simulink model "test_lineestimator_simulink"  (R2015a)
settings: Solver=ode45  StartTime=0.0  StopTime=10.0  RelTol=1e-3
undefined symbols (not defined in the file): field_x, field_y
settings Model: Creator=tzwijger  LastModifiedBy=tzwijger

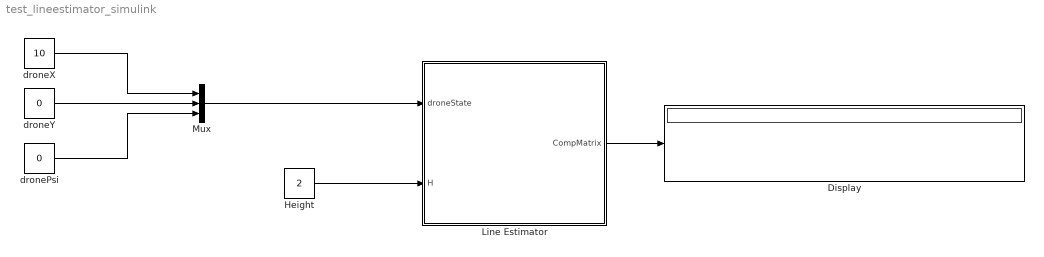
== system test_lineestimator_simulink ==
  Display : Display
  Height : Constant  Value=2
  Line Estimator : Subsystem
  Mux : Mux  Inputs=3
  dronePsi : Constant  Value=0
  droneX : Constant  Value=10
  droneY : Constant  Value=0
  wires:
  Mux/1 -> Line Estimator/1(droneState)
  droneX/1 -> Mux/1
  droneY/1 -> Mux/2
  dronePsi/1 -> Mux/3
  Height/1 -> Line Estimator/2(H)
  Line Estimator/1(CompMatrix) -> Display/1

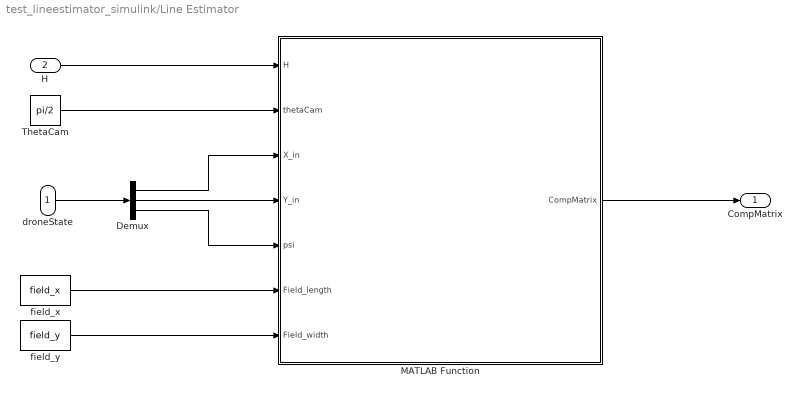
== system test_lineestimator_simulink/Line Estimator ==
  droneState : Inport
  H : Inport  Port=2
  Demux : Demux  Outputs=3
  MATLAB Function : MATLAB Function  TreatAsAtomicUnit=on
  ThetaCam : Constant  Value=pi/2
  field_x : Constant  Value=field_x
  field_y : Constant  Value=field_y
  CompMatrix : Outport
  wires:
  MATLAB Function/1(CompMatrix) -> CompMatrix/1
  ThetaCam/1 -> MATLAB Function/2(thetaCam)
  H/1 -> MATLAB Function/1(H)
  droneState/1 -> Demux/1
  Demux/1 -> MATLAB Function/3(X_in)
  Demux/2 -> MATLAB Function/4(Y_in)
  Demux/3 -> MATLAB Function/5(psi)
  field_x/1 -> MATLAB Function/6(Field_length)
  field_y/1 -> MATLAB Function/7(Field_width)

== matlab function test_lineestimator_simulink/Line Estimator/MATLAB Function ==
  data: H input; CompMatrix output; thetaCam input; X_in input; Y_in input; psi input; Field_length input; Field_width input
function CompMatrix   = World(H,thetaCam,X_in,Y_in,psi,Field_length,Field_width)

% %field line numbering:  222222222222222222223
%                         1                   3
%                         1                   3
%                         1                   3
%                         1                   3
%                         1                   3
%                         144444444444444444443

% Psi: conter-clock wise positive. zero at localization Y axis
% Theta and rho are defined according to matlab hough transform matrix

Vision=2*H*tan(thetaCam/2);
X_Vision=Vision;  %<--------------->
Y_Vision=Vision;  %|
                  %|

X=X_in-X_Vision/2;  %moving the origin from center of the camera to top left
Y=-Y_in+Y_Vision/2;
%%%%%%%%%%%%%%%%%%%%%%%%%%%%%%%%%%%%%%%%%%%%%%%%%%%%%%%%%%%%%%%%%%%%%%%%%%
%Field_length=10;   %dimentions of the field%<--------------->

%Field_width=8; %|
               %|

%%%%%%%%%%%%%%%%%%%%%%%%%%%%%%%%%%%%%%%%%%%%%%%%%%%%%%%%%%%%%%%%%%%%%%%%%%
theta1=(pi)+psi;       %calculate the theta of each side line
theta2=(-pi/2)-psi;
theta3=(0)+psi;
theta4=(pi/2)+psi;
%%%%%%%%%%%%%%%%%%%%%%%%%%%%%%%%%%%%%%%%%%%%%%%%%%%%%%%%%%%%%%%%%%%%%%%%%%%
rho1=abs(X+(Field_length)/2); %calculate rho of each side line with respect to top left cordinate
rho2=abs(Y+(Field_width)/2);
rho3= abs(-X+(Field_length)/2);
rho4= abs(-Y+(Field_width)/2);
%%%%%%%%%%%%%%%%%%%%%%%%%%%%%%%%%%%%%%%%%%%%%%%%%%%%%%%%%%%%%%%%%%%%%%%%
X1=X_in;  %having center to compare the distance and rho
Y1=-Y_in;

rho11=abs(X1+(Field_length)/2);
rho21=abs(Y1+(Field_width)/2);
rho31= abs(-X1+(Field_length)/2);
rho41= abs(-Y1+(Field_width)/2);
%%%%%%%%%%%%%%%%%%%%%%%%%%%%%%%%%%%%%%%%%%%%%%%%%%%%%%%%%%%%%%%%%%%%%%%%%%

Lines=[rho1,theta1,rho11;
rho2,theta2,rho21;
rho3,theta3,rho31;
rho4,theta4,rho41];
B=zeros(4,5);

for k=1:4
    
    i=0;
    rho=Lines(k,1);
    theta=Lines(k,2);
    %if -Y_Vision*sin(theta)<rho &&  rho<X_Vision*cos(theta)
    if Lines(k,3)<X_Vision
        i=1;
        

    end
    if theta>=(2*pi) 
        theta=theta-2*pi;
    end
    if theta<0
        theta=theta+2*pi;
    end
    B(k,:)=[k i 0 rho theta];
end
B(1,3)=2;
B(2,3)=1;
B(3,3)=2;
B(4,3)=1;

CompMatrix=B;
